simulink model "AAI_Draft"  (R2022b)
settings: Solver=FixedStepAuto  StartTime=0.0  StopTime=10.0  FixedStep=1e-3  RelTol=1e-3  EnableMultiTasking=on
undefined symbols (not defined in the file): D0, D10, D11, D12, D13, D2, D4, D5, D6, D7, D8, D9, PTA0, PTA2, PTB23, PTB9, PTC16, PTC2, PTC3, PTC4, PTD0, PTD1, PTD2, PTD3
libraries: frdmk64flib x12
settings Model: ExtModeTrigDuration=5  Creator=rebec  LastModifiedBy=rebec
settings OptimizationCC: EnhancedBackFolding=on  PassReuseOutputArgsAs=Individual arguments  ZeroExternalMemoryAtStartup=off  ZeroInternalMemoryAtStartup=off  MaxStackSize=64  OptimizeBlockOrder=speed  DifferentSizesBufferReuse=on  OptimizationCustomize=off  EfficientTunableParamExpr=on
settings DebuggingCC: ParameterTunabilityLossMsg=error
settings HardwareCC: ProdBitPerPointer=32  ProdBitPerSizeT=32  ProdBitPerPtrDiffT=32  ProdLargestAtomicInteger=Long  ProdLargestAtomicFloat=Double  ProdWordSize=32  ProdHWDeviceType=ARM Compatible->ARM Cortex
settings SFSimCC: MATLABDynamicMemAlloc=off
settings RTWCC: Description=Embedded Coder  SystemTargetFile=ert.tlc  HardwareBoard=NXP FRDM-K64F  TLCOptions="-aInlineSetEventsForThisBaseRateFcn=TLC_FALSE -aSuppressMultiTaskScheduler=TLC_FALSE  -aRateBasedStepFcn=0"  TemplateMakefile=ert_default_tmf  Toolchain=GNU Tools for ARM Embedded Processors
settings CodeAppCC: ForceParamTrailComments=on  IgnoreCustomStorageClasses=off  OperatorAnnotations=on  SimulinkDataObjDesc=on  SFDataObjDesc=on  InsertBlockDesc=on
settings ERTTargetCC: ExtModeTransport=4  ExtModeMexFile=sendToCommService

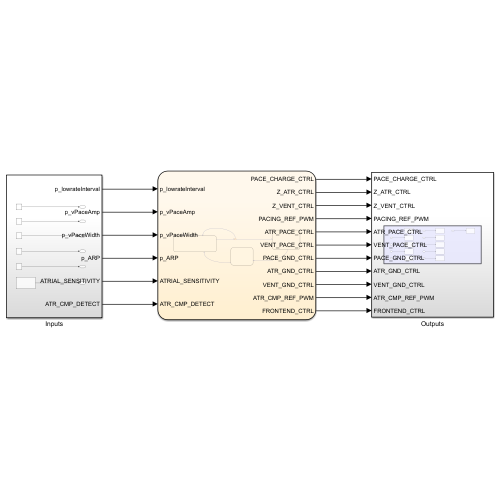
[thumbnail: Simulink's stored preview of the top-level diagram]
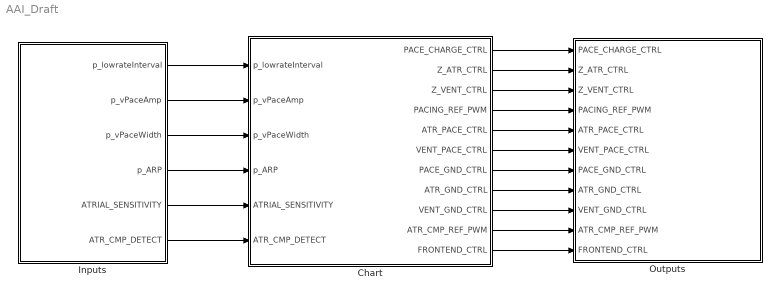
== system AAI_Draft ==
  Chart : Stateflow chart  TreatAsAtomicUnit=on
      settings: PortSchema="{\"entries\":[{\"content\":{\"sides\":[{\"content\":{\"connectorIds\":[\"In1\",\"In2\",\"In3\",\"In4\",\"In5\",\"In6\"]},\"type\":\"ConnectorPlacement.EquallySpacedRectSide\",\"uuid\":\"2be29775-b28e-43be-a3fc-e0037ad07e5c\"},{\"content\":{\"connectorIds\":[\"Out1\",\"Out2\",\"Out4\",\"Out3\",\"Out5\",\"Out6\",\"Out7\",\"Out8\",\"Out9\",\"Out11\",\"Out10\"],\"side\":\"RIGHT\"},\"type\":\"ConnectorPlacement.EquallySpacedRectSide\",\"uuid\":\"14bc2f2b-37ca-4c6e-8a62-f871f796469f\"},{\"content\":{\"connectorIds\":[],\"side\":\"TOP\"},\"type\":\"ConnectorPlacement.EquallySpacedRectSide\",\"uuid\":\"4d949104-914e-42f2-bd7c-2ab0dcae6921\"}]},\"type\":\"ConnectorPlacement.EquallySpacedConnector\",\"uuid\":\"bbaae15b-13fc-4243-8ff1-081cbec52a8c\"}],\"packageUris\":[\"http://schema.mathworks.com/mf0/Connector/R2020b\"],\"version\":\"1.0\"}"
  Inputs : Subsystem
  Outputs : Subsystem
  wires:
  Inputs/1(p_lowrateInterval) -> Chart/1(p_lowrateInterval)
  Inputs/2(p_vPaceAmp) -> Chart/2(p_vPaceAmp)
  Inputs/3(p_vPaceWidth) -> Chart/3(p_vPaceWidth)
  Inputs/4(p_ARP) -> Chart/4(p_ARP)
  Inputs/5(ATRIAL_SENSITIVITY) -> Chart/5(ATRIAL_SENSITIVITY)
  Inputs/6(ATR_CMP_DETECT) -> Chart/6(ATR_CMP_DETECT)
  Chart/1(PACE_CHARGE_CTRL) -> Outputs/1(PACE_CHARGE_CTRL)
  Chart/2(Z_ATR_CTRL) -> Outputs/2(Z_ATR_CTRL)
  Chart/3(PACING_REF_PWM) -> Outputs/4(PACING_REF_PWM)
  Chart/4(Z_VENT_CTRL) -> Outputs/3(Z_VENT_CTRL)
  Chart/10(FRONTEND_CTRL) -> Outputs/11(FRONTEND_CTRL)
  Chart/11(ATR_CMP_REF_PWM) -> Outputs/10(ATR_CMP_REF_PWM)
  Chart/9(VENT_GND_CTRL) -> Outputs/9(VENT_GND_CTRL)
  Chart/8(ATR_GND_CTRL) -> Outputs/8(ATR_GND_CTRL)
  Chart/7(PACE_GND_CTRL) -> Outputs/7(PACE_GND_CTRL)
  Chart/6(VENT_PACE_CTRL) -> Outputs/6(VENT_PACE_CTRL)
  Chart/5(ATR_PACE_CTRL) -> Outputs/5(ATR_PACE_CTRL)

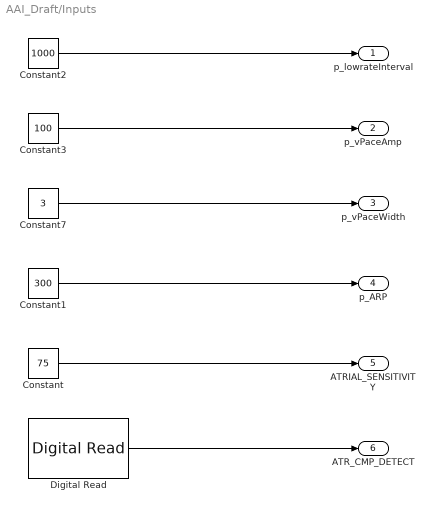
== system AAI_Draft/Inputs ==
  Constant : Constant  Value=75
  Constant1 : Constant  Value=300
  Constant2 : Constant  Value=1000
  Constant3 : Constant  Value=100
  Constant7 : Constant  Value=3
  Digital Read : frdmk64flib/Digital Read  Whichpin=PTC16 (D0)  SampleTime=-1
  p_lowrateInterval : Outport
  p_vPaceAmp : Outport  Port=2
  p_vPaceWidth : Outport  Port=3
  p_ARP : Outport  Port=4
  ATRIAL_SENSITIVITY : Outport  Port=5
  ATR_CMP_DETECT : Outport  Port=6
  wires:
  Constant3/1 -> p_vPaceAmp/1
  Constant/1 -> ATRIAL_SENSITIVITY/1
  Constant2/1 -> p_lowrateInterval/1
  Constant7/1 -> p_vPaceWidth/1
  Digital Read/1 -> ATR_CMP_DETECT/1
  Constant1/1 -> p_ARP/1

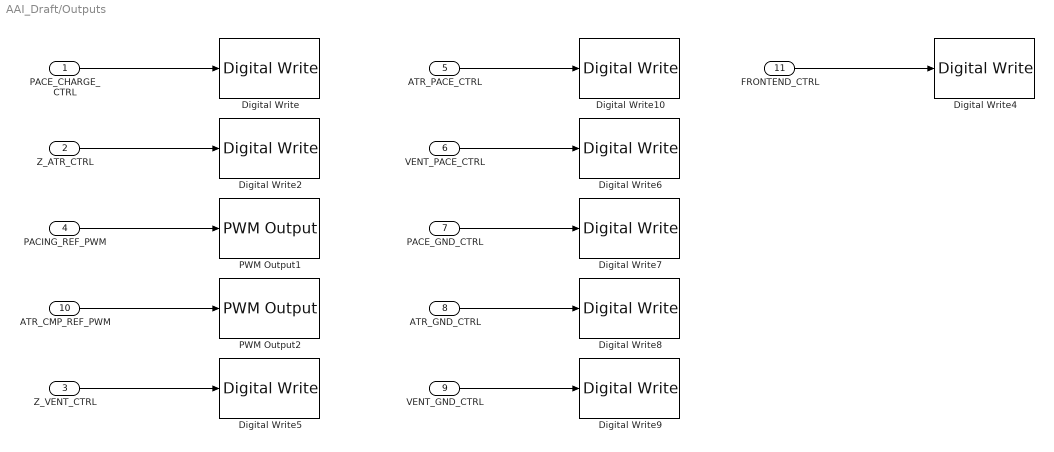
== system AAI_Draft/Outputs ==
  PACE_CHARGE_CTRL : Inport
  Z_ATR_CTRL : Inport  Port=2
  Z_VENT_CTRL : Inport  Port=3
  PACING_REF_PWM : Inport  Port=4
  ATR_PACE_CTRL : Inport  Port=5
  VENT_PACE_CTRL : Inport  Port=6
  PACE_GND_CTRL : Inport  Port=7
  ATR_GND_CTRL : Inport  Port=8
  VENT_GND_CTRL : Inport  Port=9
  ATR_CMP_REF_PWM : Inport  Port=10
  FRONTEND_CTRL : Inport  Port=11
  Digital Write : frdmk64flib/Digital Write  Whichpin=PTB9 (D2)
  Digital Write10 : frdmk64flib/Digital Write  Whichpin=PTA0 (D8)
  Digital Write2 : frdmk64flib/Digital Write  Whichpin=PTB23 (D4)
  Digital Write4 : frdmk64flib/Digital Write  Whichpin=PTD1 (D13)
  Digital Write5 : frdmk64flib/Digital Write  Whichpin=PTC3 (D7)
  Digital Write6 : frdmk64flib/Digital Write  Whichpin=PTC4 (D9)
  Digital Write7 : frdmk64flib/Digital Write  Whichpin=PTD0 (D10)
  Digital Write8 : frdmk64flib/Digital Write  Whichpin=PTD2 (D11)
  Digital Write9 : frdmk64flib/Digital Write  Whichpin=PTD3 (D12)
  PWM Output1 : frdmk64flib/PWM Output  Whichpin=PTA2 (D5)  InitialFrequency=2000  InitialDutyCycle=0
  PWM Output2 : frdmk64flib/PWM Output  Whichpin=PTC2 (D6)  InitialFrequency=2000  InitialDutyCycle=0
  wires:
  ATR_GND_CTRL/1 -> Digital Write8/1
  Z_ATR_CTRL/1 -> Digital Write2/1
  VENT_PACE_CTRL/1 -> Digital Write6/1
  PACING_REF_PWM/1 -> PWM Output1/1
  VENT_GND_CTRL/1 -> Digital Write9/1
  PACE_GND_CTRL/1 -> Digital Write7/1
  FRONTEND_CTRL/1 -> Digital Write4/1
  PACE_CHARGE_CTRL/1 -> Digital Write/1
  Z_VENT_CTRL/1 -> Digital Write5/1
  ATR_CMP_REF_PWM/1 -> PWM Output2/1
  ATR_PACE_CTRL/1 -> Digital Write10/1

== stateflow chart AAI_Draft/Chart ==
  state Pacing
    entry:
    PACE_CHARGE_CTRL = 0;
    PACE_GND_CTRL = 1;
    ATR_PACE_CTRL = 1;
    ATR_GND_CTRL = 0;
    Z_ATR_CTRL = 0;
    Z_VENT_CTRL = 0;
    VENT_GND_CTRL = 0;
    VENT_PACE_CTRL = 0;
  state Charging
    entry:
    PACING_REF_PWM = p_vPaceAmp;
    FRONTEND_CTRL = 1;
    ATR_CMP_REF_PWM = ATRIAL_SENSITIVITY;
    PACE_CHARGE_CTRL = 1;
    VENT_PACE_CTRL = 0;
    ATR_PACE_CTRL = 0;
  state Discharging
    entry:
    PACE_GND_CTRL = 1;
    VENT_PACE_CTRL = 0;
    ATR_PACE_CTRL = 0;
    Z_ATR_CTRL = 0;
    Z_VENT_CTRL = 0;
    ATR_GND_CTRL = 1;
    VENT_GND_CTRL = 0;
  (junction 43) -> Charging [order 1] : [ATR_CMP_DETECT == 1]
  (default) -> Charging
  Charging -> (junction 43) : after(p_ARP, msec)
  (junction 43) -> Pacing [order 2] : after(p_lowrateInterval, msec)
  Pacing -> Discharging : after(p_vPaceWidth, msec)
  Discharging -> Charging
  data: PACE_CHARGE_CTRL output int16; Z_ATR_CTRL output int16; PACING_REF_PWM output double; Z_VENT_CTRL output int16; ATR_PACE_CTRL output int16; VENT_PACE_CTRL output int16; PACE_GND_CTRL output int16; ATR_GND_CTRL output int16; VENT_GND_CTRL output int16; p_lowrateInterval input; p_vPaceAmp input; p_vPaceWidth input; p_ARP input; ATRIAL_SENSITIVITY input; ATR_CMP_DETECT input; FRONTEND_CTRL output; ATR_CMP_REF_PWM output
